simulink model "untitled"  (R2021a)
settings: Solver=VariableStepAuto  StartTime=0.0  StopTime=inf  RelTol=1e-3
libraries: mobileRoboticsLib x4, simulink_extras x3
settings Model: Creator=its_ghani  LastModifiedBy=its_ghani

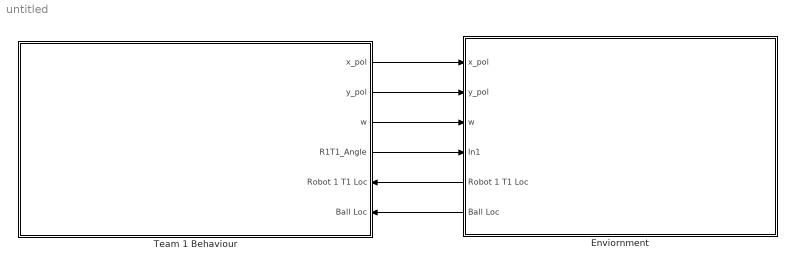
== system untitled ==
  Enviornment : Subsystem
      settings: PortSchema="{\"entries\":[{\"content\":{\"sides\":[{\"content\":{\"connectorIds\":[\"In1\",\"In2\",\"In3\",\"In4\",\"Out1\",\"Out2\"]},\"type\":\"ConnectorPlacement.EquallySpacedRectSide\",\"uuid\":\"bfc4f995-18bb-40a5-813e-439d500b4bf9\"},{\"content\":{\"connectorIds\":[],\"side\":\"RIGHT\"},\"type\":\"ConnectorPlacement.EquallySpacedRectSide\",\"uuid\":\"3fb6b8a6-16df-4a59-8ba5-6321e26d1fdd\"},{\"content\":{\"connectorIds\":[],\"side\":\"TOP\"},\"type\":\"ConnectorPlacement.EquallySpacedRectSide\",\"uuid\":\"a9e4cd1b-3afe-4395-99fa-15aef12a4070\"}]},\"type\":\"ConnectorPlacement.EquallySpacedConnector\",\"uuid\":\"a6ca697e-fe67-43ac-b669-91f3e6c836c9\"}],\"packageUris\":[\"http://schema.mathworks.com/mf0/Connector/R2020b\"],\"version\":\"1.0\"}"
  Team 1 Behaviour : Subsystem
      settings: PortSchema="{\"entries\":[{\"content\":{\"sides\":[{\"content\":{\"connectorIds\":[]},\"type\":\"ConnectorPlacement.EquallySpacedRectSide\",\"uuid\":\"be901545-21b9-45e5-bac5-a8cb9027aef5\"},{\"content\":{\"connectorIds\":[\"Out1\",\"Out2\",\"Out3\",\"Out4\",\"In1\",\"In2\"],\"side\":\"RIGHT\"},\"type\":\"ConnectorPlacement.EquallySpacedRectSide\",\"uuid\":\"b7c1eb84-2f14-4c7f-a74c-d56efbe0743e\"},{\"content\":{\"connectorIds\":[],\"side\":\"TOP\"},\"type\":\"ConnectorPlacement.EquallySpacedRectSide\",\"uuid\":\"aca41723-ed3f-4bd2-8fc1-457d075e3460\"}]},\"type\":\"ConnectorPlacement.EquallySpacedConnector\",\"uuid\":\"e10e22f1-c8f0-4dfc-85d2-4ba01528372d\"}],\"packageUris\":[\"http://schema.mathworks.com/mf0/Connector/R2020b\"],\"version\":\"1.0\"}"
  wires:
  Team 1 Behaviour/4("R1T1_Angle\t") -> Enviornment/4(In1)
  Enviornment/1(Robot 1 T1 Loc) -> Team 1 Behaviour/1(Robot 1 T1 Loc)
  Enviornment/2(Ball Loc) -> Team 1 Behaviour/2(Ball Loc)
  Team 1 Behaviour/1(x_pol) -> Enviornment/1(x_pol)
  Team 1 Behaviour/2(y_pol) -> Enviornment/2(y_pol)
  Team 1 Behaviour/3(w) -> Enviornment/3(w)

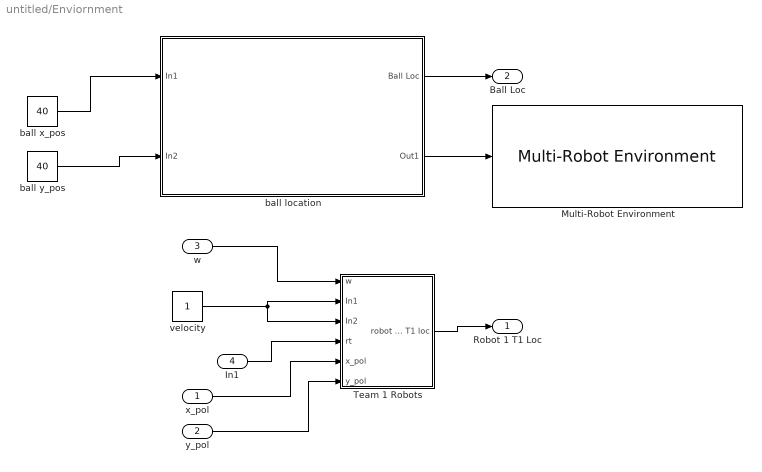
== system untitled/Enviornment ==
  x_pol : Inport
  y_pol : Inport  Port=2
  w : Inport  Port=3
  In1 : Inport  Port=4
  "\tTeam 1 Robots" : Subsystem
  Multi-Robot Environment : mobileRoboticsLib/Environments/Multi-Robot Environment  numRobots=1  showWaypoints=off  showObjects=on  objectColors=[1 0 0;0 1 0;0 0 1]  objectMarkers='s'  showRobotIds=on  plotSensorLines=off
      settings: SourceProductName=Mobile Robotics Simulation Toolbox
  ball location : Subsystem
  ball x_pos : Constant  Value=40
  ball y_pos : Constant  Value=40
  velocity : Constant
  Robot 1 T1 Loc : Outport
  Ball Loc : Outport  Port=2
  wires:
  ball x_pos/1 -> ball location/1(In1)
  ball y_pos/1 -> ball location/2(In2)
  ball location/2(Out1) -> Multi-Robot Environment/1
  "\tTeam 1 Robots"/1(robot 1 T1 loc) -> Robot 1 T1 Loc/1
  ball location/1(Ball Loc) -> Ball Loc/1
  In1/1 -> "\tTeam 1 Robots"/4(rt)
  velocity/1 -> "\tTeam 1 Robots"/3(In2), "\tTeam 1 Robots"/2(In1)
  x_pol/1 -> "\tTeam 1 Robots"/5(x_pol)
  y_pol/1 -> "\tTeam 1 Robots"/6(y_pol)
  w/1 -> "\tTeam 1 Robots"/1(w)

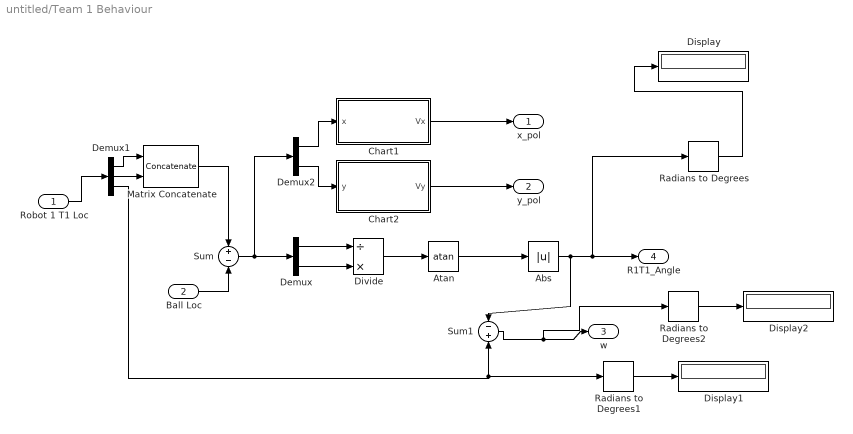
== system untitled/Team 1 Behaviour ==
  Robot 1 T1 Loc : Inport
  Ball Loc : Inport  Port=2
  Abs : Abs
  Atan : Trigonometry  Operator=atan
  Chart1 : Stateflow chart  TreatAsAtomicUnit=on
  Chart2 : Stateflow chart  TreatAsAtomicUnit=on
  Demux : Demux  Outputs=2
  Demux1 : Demux  Outputs=3
  Demux2 : Demux  Outputs=2
  Display : Display
  Display1 : Display
  Display2 : Display
  Divide : Product  Inputs=/*
  Matrix Concatenate : Concatenate  Mode=Multidimensional array  ConcatenateDimension=2
  Radians to Degrees : simulink_extras/Transformations/Radians to Degrees
  Radians to Degrees1 : simulink_extras/Transformations/Radians to Degrees
  Radians to Degrees2 : simulink_extras/Transformations/Radians to Degrees
  Sum : Sum  Inputs=+-
  Sum1 : Sum  Inputs=-+
  x_pol : Outport
  y_pol : Outport  Port=2
  w : Outport  Port=3
  "R1T1_Angle\t" : Outport  Port=4
  wires:
  Ball Loc/1 -> Sum/2
  Sum/1 -> Demux2/1, Demux/1
  Divide/1 -> Atan/1
  Robot 1 T1 Loc/1 -> Demux1/1
  Demux1/1 -> Matrix Concatenate/1
  Demux1/2 -> Matrix Concatenate/2
  Matrix Concatenate/1 -> Sum/1
  Demux/1 -> Divide/1
  Demux/2 -> Divide/2
  Demux2/2 -> Chart2/1(y)
  Chart1/1(Vx) -> x_pol/1
  Chart2/1(Vy) -> y_pol/1
  Atan/1 -> Abs/1
  Abs/1 -> Sum1/1, Radians to Degrees/1, "R1T1_Angle\t"/1
  Demux2/1 -> Chart1/1(x)
  Demux1/3 -> Radians to Degrees1/1, Sum1/2
  Sum1/1 -> Radians to Degrees2/1, w/1
  Radians to Degrees/1 -> Display/1
  Radians to Degrees1/1 -> Display1/1
  Radians to Degrees2/1 -> Display2/1

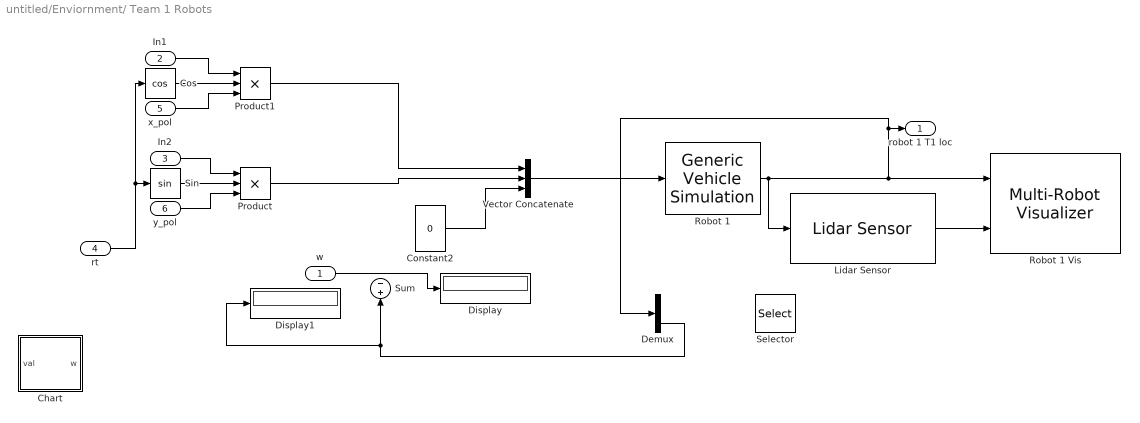
== system untitled/Enviornment/	Team 1 Robots ==
  w : Inport
  In1 : Inport  Port=2
  In2 : Inport  Port=3
  rt : Inport  Port=4
  x_pol : Inport  Port=5
  y_pol : Inport  Port=6
  Chart : Stateflow chart  TreatAsAtomicUnit=on
  Constant2 : Constant  Value=0
  Cos : Trigonometry  Operator=cos
  Demux : Demux  Outputs=3
  Display : Display
  Display1 : Display
  Lidar Sensor : mobileRoboticsLib/Environments/Lidar Sensor  sensorOffset=[ 0, 0 ]  scanAngles=[ -pi/4, 0, pi/4 ]  maxRange=5  isMultiRobot=on  robotIdx=1
      settings: SourceProductName=Mobile Robotics Simulation Toolbox
  Product : Product  Inputs=3
  Product1 : Product  Inputs=3
  Robot 1 : mobileRoboticsLib/Utilities/Generic Vehicle Simulation  initX=0  initY=0  initAngle=0  Ts=0.05
      settings: SourceProductName=Mobile Robotics Simulation Toolbox
  Robot 1 Vis : mobileRoboticsLib/Environments/Multi-Robot Visualizer  idx=1  radius=0.1  robotColor=[0 0 1]  showTraj=on  hasLidar=on  sensorOffset=[0,0]  scanAngles=[-pi/4, 0, pi/4]  hasObjDetector=off  objDetectorOffset=[0,0]  objDetectorAngle=0  objDetectorFOV=pi/3  objDetectorMaxRange=5
      settings: SourceProductName=Mobile Robotics Simulation Toolbox
  Selector : Selector  InputPortWidth=5  IndexOptions=Index vector (dialog)  Indices=[1 3]  OutputSizes=1
  Sin : Trigonometry
  Sum : Sum  Inputs=-+
  Vector Concatenate : Concatenate  NumInputs=3
  robot 1 T1 loc : Outport
  wires:
  Vector Concatenate/1 -> Robot 1/1
  Robot 1/1 -> Demux/1, robot 1 T1 loc/1, Robot 1 Vis/1, Lidar Sensor/1
  Lidar Sensor/1 -> Robot 1 Vis/2
  rt/1 -> Cos/1, Sin/1
  Sin/1 -> Product/2
  In2/1 -> Product/1
  Cos/1 -> Product1/2
  In1/1 -> Product1/1
  x_pol/1 -> Product1/3
  y_pol/1 -> Product/3
  Demux/3 -> Display1/1, Sum/2
  w/1 -> Display/1
  Constant2/1 -> Vector Concatenate/3
  Product1/1 -> Vector Concatenate/1
  Product/1 -> Vector Concatenate/2

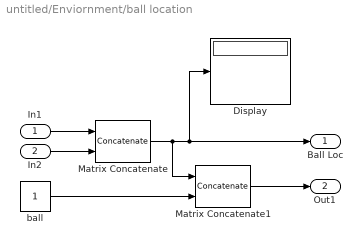
== system untitled/Enviornment/ball location ==
  In1 : Inport
  In2 : Inport  Port=2
  Display : Display
  Matrix Concatenate : Concatenate  Mode=Multidimensional array  ConcatenateDimension=2
  Matrix Concatenate1 : Concatenate  Mode=Multidimensional array  ConcatenateDimension=2
  ball : Constant
  Ball Loc : Outport
  Out1 : Outport  Port=2
  wires:
  ball/1 -> Matrix Concatenate1/2
  In1/1 -> Matrix Concatenate/1
  In2/1 -> Matrix Concatenate/2
  Matrix Concatenate/1 -> Matrix Concatenate1/1, Display/1, Ball Loc/1
  Matrix Concatenate1/1 -> Out1/1

== stateflow chart untitled/Team 1 Behaviour/Chart1 ==
  state x_pos
    du:
    Vx = 1
  state x_neg
    du:
    Vx = -1
  (default) -> x_pos
  x_pos -> x_neg : [x > 0]
  x_neg -> x_pos : [x<1]
  data: Vx output; x input

== stateflow chart untitled/Team 1 Behaviour/Chart2 ==
  state y_pos
    du:
    Vy = 1
  state y_neg
    du:
    Vy = -1
  (default) -> y_pos
  y_pos -> y_neg : [y > 0]
  y_neg -> y_pos : [y<1]
  data: y input; Vy output

== stateflow chart untitled/Enviornment/	Team 1 Robots/Chart ==
  (default) -> (junction 1)
  (junction 1) -> (junction 3) : {w=0}
  (junction 3) -> (junction 4) : {w=val}
  data: w output; val input
